simulink model "trestres"  (R2015a)
settings: Solver=ode45  StartTime=0.0  StopTime=1000.0  RelTol=1e-3
values from neighbouring files (symbols this model uses):
  k2 = 10    [20181030_1937.mat]
  p = 0.01    [20181030_1937.mat]
settings Model: Creator=Alunos  LastModifiedBy=Alunos

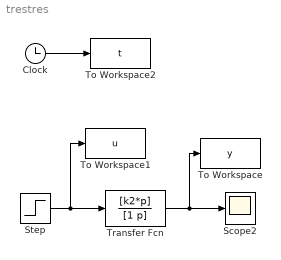
== system trestres ==
  Clock : Clock
  Scope2 : Scope
  Step : Step  SampleTime=0
  To Workspace : ToWorkspace  VariableName=y  SampleTime=-1
  To Workspace1 : ToWorkspace  VariableName=u  SampleTime=-1
  To Workspace2 : ToWorkspace  VariableName=t  SampleTime=-1
  Transfer Fcn : TransferFcn  Numerator=[k2*p]  Denominator=[1 p]
  wires:
  Step/1 -> To Workspace1/1, Transfer Fcn/1
  Transfer Fcn/1 -> To Workspace/1, Scope2/1
  Clock/1 -> To Workspace2/1
